simulink model "APT_Receiver"  (R2024b)
settings: Solver=VariableStepAuto  StartTime=0.0  StopTime=540  RelTol=1e-3
undefined symbols (not defined in the file or in its folder): designMultirateFIR
libraries: matrix_library x2, dspfdesign x1, dspmlti4 x1, dspvision x1, dspsrcs4 x1
Description:
  | % APT_Receiver: This model demodulate the APT signal
  | % Copyright (C) 2025  Mohammad Safa
  | % GitHub Repository: https://github.com/mhr98/APT-Receiver
  | %
  | % This program is free software: you can redistribute it and/or modify
  | % it under the terms of the GNU General Public License as published by
  | % the Free Software Foundation, either version 3 of the License, or
  | % (at your option) any later version.
  | %
  | % This program is distributed in the hope that it will be useful,
  | % but WITHOUT ANY WARRANTY; without even the implied warranty of
  | % MERCHANTABILITY or FITNESS FOR A PARTICULAR PURPOSE.  See the
  | % GNU General Public License for more details.
  | %
  | % You should have received a copy of the GNU General Public License
  | % along with this program.  If not, see <https://www.gnu.org/licenses/>.
settings Model: Creator=ASUS  LastModifiedBy=ASUS

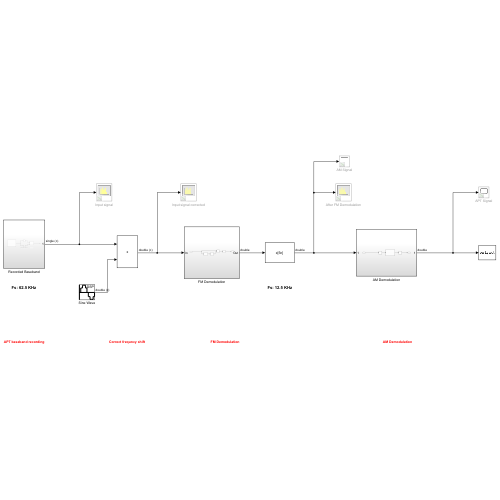
[thumbnail: Simulink's stored preview of the top-level diagram]
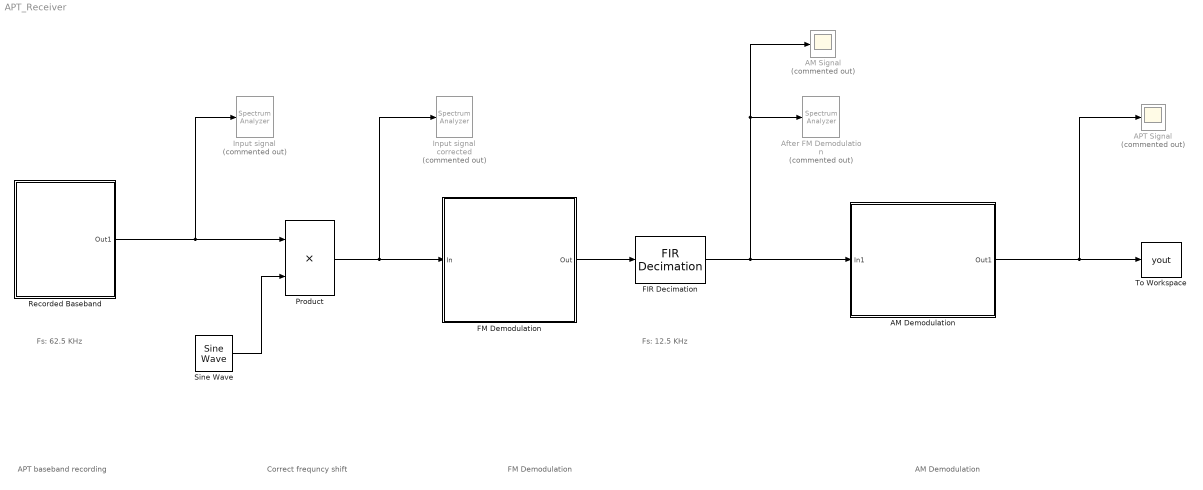
== system APT_Receiver ==
  note: APT baseband recording
  note: Fs: 62.5 KHz
  note: Fs: 12.5 KHz
  note: Correct frequncy shift
  note: FM Demodulation
  note: AM Demodulation
  AM Demodulation : Subsystem
  AM Signal : Scope  Commented=on
  APT Signal : Scope  Commented=on
  After FM Demodulation : SpectrumAnalyzer  Commented=on  WindowPosition=[-75.000000,129.000000,800.000000,500.000000,]  ScopeFrameLocation=window  Method=Welch  FrequencyResolutionMethod=Window length  WindowInvariantSamplesPerUpdate=on  WindowLength=4096  YLimits=[-53.5778662,29.95807722]  SelectedToolstripTab=spectrumAnalyzerToolstrip.estimationTab
  FIR Decimation : dspmlti4/FIR Decimation  FilterSource=Auto  h=designMultirateFIR(1,2)  D=5  filtStruct=Direct form  FilterObject=FDECIM  InputProcessing=Columns as channels (frame based)  framing=Allow multirate processing  AllowArbitraryInputLength=off  inputOffset=0  outputBufInitCond=0  roundingMode=Floor  overflowMode=off  firstCoeffDataTypeStr=Inherit: Same word length as input  firstCoeffMin=[]  firstCoeffMax=[]  firstCoeffLastDataTypeStr=Inherit: Same word length as input  outputDataTypeStr=Inherit: Same as accumulator  outputMin=[]  outputMax=[]  outputLastDataTypeStr=Inherit: Same as accumulator
  FM Demodulation : Subsystem
  Input signal : SpectrumAnalyzer  Commented=on  WindowPosition=[368.000000,182.000000,800.000000,500.000000,]  ScopeFrameLocation=window  WindowInvariantSamplesPerUpdate=on  YLimits=[-65.71776474,-14.50527088]
  Input signal corrected : SpectrumAnalyzer  Commented=on  WindowPosition=[368.000000,182.000000,800.000000,500.000000,]  ScopeFrameLocation=window  WindowInvariantSamplesPerUpdate=on  YLimits=[-65.71776474,-14.50527088]
  Product : Product
  Recorded Baseband : Subsystem
  Sine Wave : dspsrcs4/Sine Wave  Amplitude=1  Frequency=-3.2e3  Phase=0  SampleMode=Discrete  OutComplex=Complex  CompMethod=Trigonometric fcn  TableSize=Speed  SampleTime=1/62.5e3  SamplesPerFrame=4096  ResetState=Restart at time zero  OutputFrames=off  dataType=double  wordLen=16  udDataType=sfix(16)  fracBitsMode=Best precision  numFracBits=15  OutDataTypeStr=double  LastOutDataTypeStr=double
  To Workspace : ToWorkspace  VariableName=yout  SampleTime=-1
      settings: Save2DSignal=2-D array (concatenate along first dimension)
  wires:
  FM Demodulation/1(Out) -> FIR Decimation/1
  FIR Decimation/1 -> AM Signal/1, After FM Demodulation/1, AM Demodulation/1(In1)
  Sine Wave/1 -> Product/2
  Recorded Baseband/1(Out1) -> Input signal/1, Product/1
  Product/1 -> FM Demodulation/1(In), Input signal corrected/1
  AM Demodulation/1(Out1) -> APT Signal/1, To Workspace/1

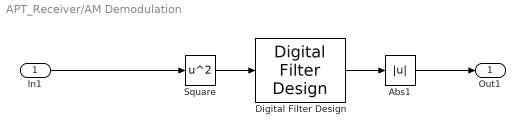
== system APT_Receiver/AM Demodulation ==
  In1 : Inport
  Abs1 : Abs  SaturateOnIntegerOverflow=off
  Digital Filter Design : dspfdesign/Digital Filter Design  mwdsp_browser_bugfix_var=off
  Square : Math  Operator=square  SignedPower=on
  Out1 : Outport
  wires:
  Digital Filter Design/1 -> Abs1/1
  Abs1/1 -> Out1/1
  Square/1 -> Digital Filter Design/1
  In1/1 -> Square/1

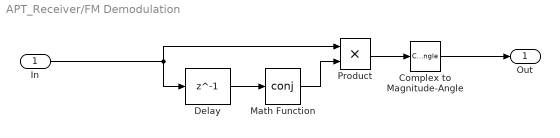
== system APT_Receiver/FM Demodulation ==
  In : Inport
  Complex to Magnitude-Angle : ComplexToMagnitudeAngle  Output=Angle
  Delay : Delay  DelayLength=1  InputProcessing=Columns as channels (frame based)
  Math Function : Math  Operator=conj
  Product : Product
  Out : Outport
  wires:
  In/1 -> Delay/1, Product/1
  Delay/1 -> Math Function/1
  Math Function/1 -> Product/2
  Complex to Magnitude-Angle/1 -> Out/1
  Product/1 -> Complex to Magnitude-Angle/1

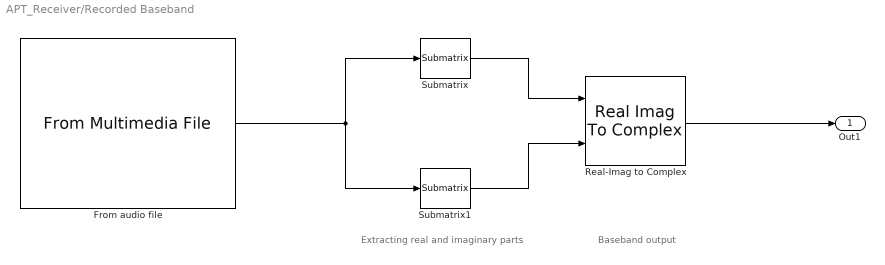
== system APT_Receiver/Recorded Baseband ==
  note: Baseband output
  note: Extracting real and imaginary parts
  From audio file : dspvision/From Multimedia File  inputFilename=D:\My Courses\noaa_satellite\final\apt_signal.wav  readRange=[1 Inf]  loop=on  numPlays=inf  outputStreams=Audio only  videoDataType=single  audioDataType=single  inheritSampleTime=on  userDefinedSampleTime=1/30  noAudioOutput=off  isIntensityVideo=off  fourcc=RGB  colorVideoFormat=One multidimensional signal  outputEOF=off  dataOrg=Column-major  audioFrameSize=4096  computeAudioFrameSize=off  outSamplingMode=Sample based
  Real-Imag to Complex : RealImagToComplex
  Submatrix : matrix_library/Submatrix  RowSpan=All rows  RowStartMode=First  RowStartIndex=1  RowEndMode=Last  RowEndIndex=1  ColSpan=One column  ColStartMode=First  ColStartIndex=1  ColEndMode=Last  ColEndIndex=1
  Submatrix1 : matrix_library/Submatrix  RowSpan=All rows  RowStartMode=First  RowStartIndex=1  RowEndMode=Last  RowEndIndex=1  ColSpan=One column  ColStartMode=Last  ColStartIndex=1  ColEndMode=Last  ColEndIndex=1
  Out1 : Outport
  wires:
  Submatrix1/1 -> Real-Imag to Complex/2
  From audio file/1 -> Submatrix1/1, Submatrix/1
  Submatrix/1 -> Real-Imag to Complex/1
  Real-Imag to Complex/1 -> Out1/1
